simulink model "Transformer_example"  (R2016b)
settings: Solver=VariableStepAuto  StartTime=0.0  StopTime=1000  RelTol=1e-3
InitFcn:
  | d1=1;
  | d2=1;
  | d3=3;
  | d4=3;
  | tau=1000000000000
undefined symbols (not defined in the file): d10, d9
libraries: simulink x1
settings Model: Creator=SHAAD  LastModifiedBy=SHAAD

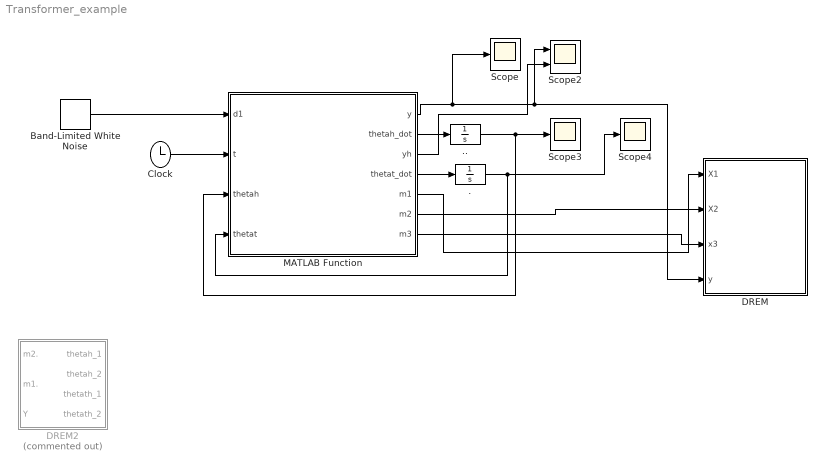
== system Transformer_example ==
  . : Integrator  InitialCondition=[1 2 3]
  .. : Integrator
  Band-Limited White Noise : simulink/Sources/Band-Limited White Noise  Cov=[0.001]  Ts=0.1  seed=[23341]
  Clock : Clock
  DREM : Subsystem
  DREM2 : Subsystem  Commented=on
  MATLAB Function : MATLAB Function  TreatAsAtomicUnit=on
  Scope : Scope
  Scope2 : Scope  NumInputPorts=2
  Scope3 : Scope
  Scope4 : Scope
  wires:
  Clock/1 -> MATLAB Function/2(t)
  MATLAB Function/2(thetah_dot) -> ../1
  ../1 -> MATLAB Function/3(thetah), Scope3/1
  MATLAB Function/4(thetat_dot) -> ./1
  ./1 -> Scope4/1, MATLAB Function/4(thetat)
  MATLAB Function/3(yh) -> Scope2/2
  MATLAB Function/5(m1) -> DREM/1(X1)
  MATLAB Function/6(m2) -> DREM/2(X2)
  MATLAB Function/1(y) -> Scope/1, DREM/4(y), Scope2/1
  MATLAB Function/7(m3) -> DREM/3(x3)
  Band-Limited White Noise/1 -> MATLAB Function/1(d1)

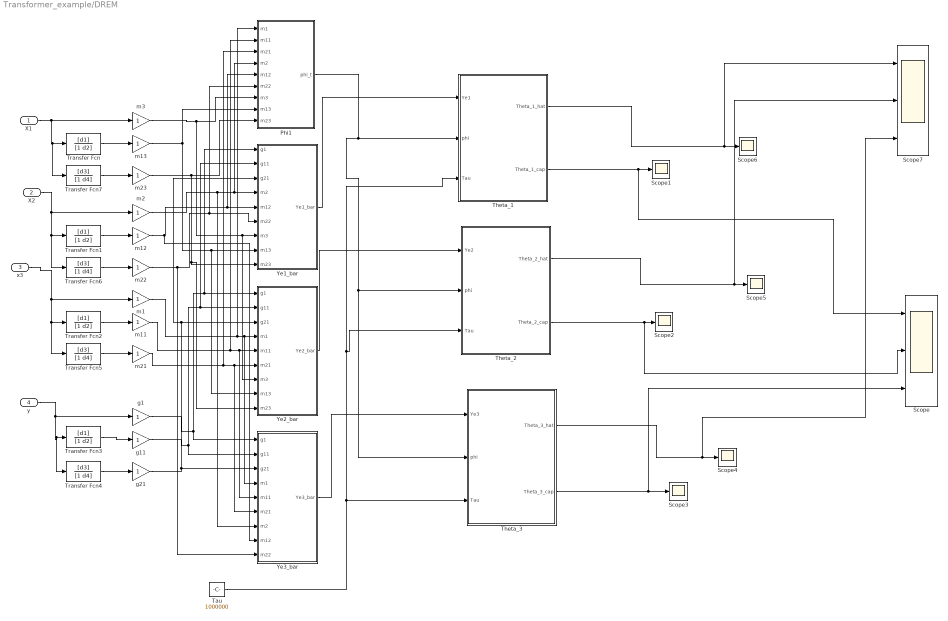
== system Transformer_example/DREM ==
  X1 : Inport
  X2 : Inport  Port=2
  x3 : Inport  Port=3
  y : Inport  Port=4
  Phi1 : Subsystem
  Scope : Scope  NumInputPorts=3
  Scope{1..6} (6 alike) : Scope
  Scope7 : Scope  NumInputPorts=3
  Tau : Constant  Value=1000000  SampleTime=-1
  Theta_1 : Subsystem
  Theta_2 : Subsystem
  Theta_3 : Subsystem
  Transfer Fcn{,1..3} (4 alike) : TransferFcn  Numerator=[d1]  Denominator=[1 d2]
  Transfer Fcn{4..7} (4 alike) : TransferFcn  Numerator=[d3]  Denominator=[1 d4]
  Ye1_bar : Subsystem
  Ye2_bar : Subsystem
  "Ye3_bar " : Subsystem
  g1 : Gain
  g11 : Gain
  g21 : Gain
  m{1..3,11..13,21..23} (9 alike) : Gain
  wires:
  Transfer Fcn/1 -> m13/1
  X1/1 -> m3/1, Transfer Fcn7/1, Transfer Fcn/1
  Transfer Fcn7/1 -> m23/1
  Transfer Fcn1/1 -> m12/1
  X2/1 -> m2/1, Transfer Fcn6/1, Transfer Fcn1/1
  Transfer Fcn6/1 -> m22/1
  x3/1 -> m1/1, Transfer Fcn5/1, Transfer Fcn2/1
  Transfer Fcn5/1 -> m21/1
  Transfer Fcn3/1 -> g11/1
  y/1 -> Transfer Fcn4/1, Transfer Fcn3/1, g1/1
  Transfer Fcn4/1 -> g21/1
  Ye1_bar/1(Ye1_bar) -> Theta_1/1(Ye1)
  Ye2_bar/1(Ye2_bar) -> Theta_2/1(Ye2)
  Phi1/1(phi_t) -> Theta_3/2(phi), Theta_2/2(phi), Theta_1/2(phi)
  Tau/1 -> Theta_3/3(Tau), Theta_2/3(Tau), Theta_1/3(Tau)
  "Ye3_bar "/1(Ye3_bar) -> Theta_3/1(Ye3)
  g1/1 -> Ye1_bar/1(g1), Ye2_bar/1(g1), "Ye3_bar "/1(g1)
  g21/1 -> Ye2_bar/3(g21), Ye1_bar/3(g21), "Ye3_bar "/3(g21)
  m1/1 -> Phi1/1(m1), "Ye3_bar "/4(m1), Ye2_bar/4(m1)
  m11/1 -> Phi1/2(m11), "Ye3_bar "/5(m11), Ye2_bar/5(m11)
  m21/1 -> Phi1/3(m21), "Ye3_bar "/6(m21), Ye2_bar/6(m21)
  m2/1 -> "Ye3_bar "/7(m2), Ye1_bar/4(m2), Phi1/4(m2)
  m12/1 -> "Ye3_bar "/8(m12), Phi1/5(m12), Ye1_bar/5(m12)
  m22/1 -> "Ye3_bar "/9(m22), Ye1_bar/6(m22), Phi1/6(m22)
  m3/1 -> Phi1/7(m3), Ye1_bar/7(m3), Ye2_bar/7(m3)
  m13/1 -> Ye2_bar/8(m13), Ye1_bar/8(m13), Phi1/8(m13)
  m23/1 -> Phi1/9(m23), Ye2_bar/9(m23), Ye1_bar/9(m23)
  Theta_1/1(Theta_1_hat) -> Scope7/1, Scope6/1
  Theta_1/2(Theta_1_cap) -> Scope/1, Scope1/1
  Theta_2/1(Theta_2_hat) -> Scope7/2, Scope5/1
  Theta_2/2(Theta_2_cap) -> Scope/2, Scope2/1
  Theta_3/1(Theta_3_hat) -> Scope7/3, Scope4/1
  Theta_3/2(Theta_3_cap) -> Scope/3, Scope3/1
  Transfer Fcn2/1 -> m11/1
  g11/1 -> Ye1_bar/2(g11), Ye2_bar/2(g11), "Ye3_bar "/2(g11)

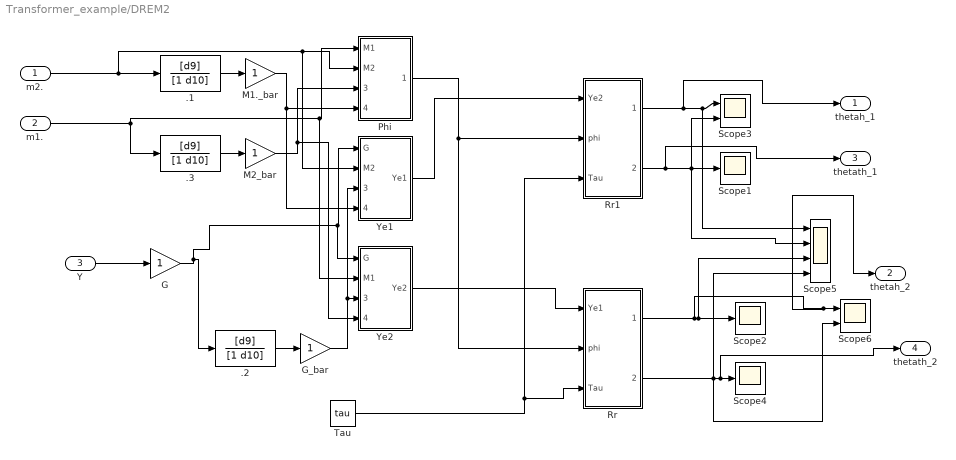
== system Transformer_example/DREM2 ==
  m2. : Inport
  m1. : Inport  Port=2
  Y : Inport  Port=3
  .1 : TransferFcn  Numerator=[d9]  Denominator=[1 d10]
  .2 : TransferFcn  Numerator=[d9]  Denominator=[1 d10]
  .3 : TransferFcn  Numerator=[d9]  Denominator=[1 d10]
  G : Gain
  G_bar : Gain
  M1._bar : Gain
  M2_bar : Gain
  Phi : Subsystem
  Rr : Subsystem
  Rr1 : Subsystem
  Scope1 : Scope
  Scope2 : Scope
  Scope3 : Scope  NumInputPorts=2
  Scope4 : Scope
  Scope5 : Scope  NumInputPorts=4
  Scope6 : Scope  NumInputPorts=2
  Tau : Constant  Value=tau  SampleTime=-1
  Ye1 : Subsystem
  Ye2 : Subsystem
  thetah_1 : Outport
  thetah_2 : Outport  Port=2
  thetath_1 : Outport  Port=3
  thetath_2 : Outport  Port=4
  wires:
  G/1 -> .2/1, Ye2/1(G), Ye1/1(G)
  Tau/1 -> Rr1/3(Tau), Rr/3(Tau)
  Y/1 -> G/1
  .2/1 -> G_bar/1
  .3/1 -> M2_bar/1
  G_bar/1 -> Ye2/3(G_bar), Ye1/3(G_bar)
  Phi/1(phi_t) -> Rr1/2(phi), Rr/2(phi)
  Rr1/2(Rr_cap) -> thetath_1/1, Scope3/2, Scope5/2, Scope1/1
  Rr/1(Rs_hat) -> thetah_2/1, Scope6/1, Scope5/3, Scope2/1
  .1/1 -> M1._bar/1
  Rr1/1(Rr_hat) -> thetah_1/1, Scope5/1, Scope3/1
  m1./1 -> Ye2/2(M1), Phi/1(M1), .3/1
  Ye1/1(Ye1) -> Rr1/1(Ye2)
  Ye2/1(Ye2) -> Rr/1(Ye1)
  M2_bar/1 -> Ye2/4("M1_bar "), Phi/3(M1_bar)
  M1._bar/1 -> Phi/4(M2_bar), Ye1/4(M2_bar)
  m2./1 -> Ye1/2(M2), Phi/2(M2), .1/1
  Rr/2(Rs_cap) -> Scope5/4, Scope6/2, thetath_2/1, Scope4/1

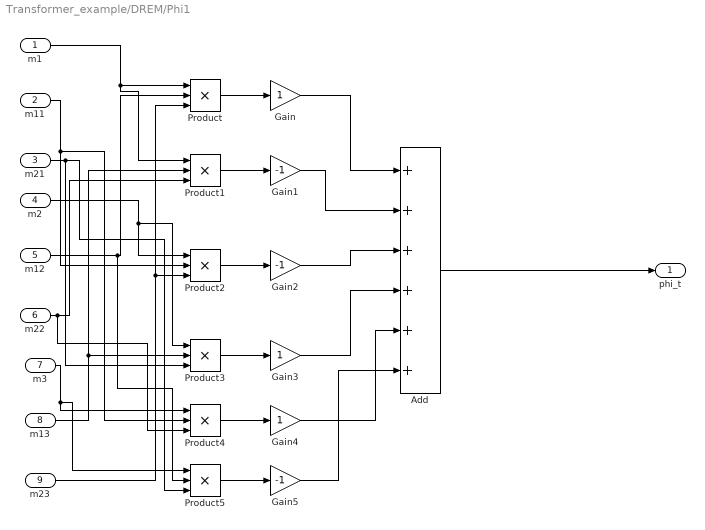
== system Transformer_example/DREM/Phi1 ==
  m1 : Inport
  m11 : Inport  Port=2
  m21 : Inport  Port=3
  m2 : Inport  Port=4
  m12 : Inport  Port=5
  m22 : Inport  Port=6
  m3 : Inport  Port=7
  m13 : Inport  Port=8
  m23 : Inport  Port=9
  Add : Sum  Inputs=++++++
  Gain : Gain
  Gain1 : Gain  Gain=-1
  Gain2 : Gain  Gain=-1
  Gain3 : Gain
  Gain4 : Gain
  Gain5 : Gain  Gain=-1
  Product{,1..5} (6 alike) : Product  Inputs=3
  phi_t : Outport
  wires:
  m1/1 -> Product1/1, Product/1
  m23/1 -> Product2/3, Product/3
  m13/1 -> Product3/2, Product1/2
  m22/1 -> Product4/3, Product1/3
  m2/1 -> Product3/1, Product2/1
  m11/1 -> Product4/2, Product2/2
  m3/1 -> Product5/1, Product4/1
  m12/1 -> Product5/2, Product/2
  m21/1 -> Product5/3, Product3/3
  Product/1 -> Gain/1
  Product1/1 -> Gain1/1
  Product2/1 -> Gain2/1
  Product3/1 -> Gain3/1
  Product4/1 -> Gain4/1
  Product5/1 -> Gain5/1
  Add/1 -> phi_t/1
  Gain/1 -> Add/1
  Gain1/1 -> Add/2
  Gain2/1 -> Add/3
  Gain3/1 -> Add/4
  Gain4/1 -> Add/5
  Gain5/1 -> Add/6

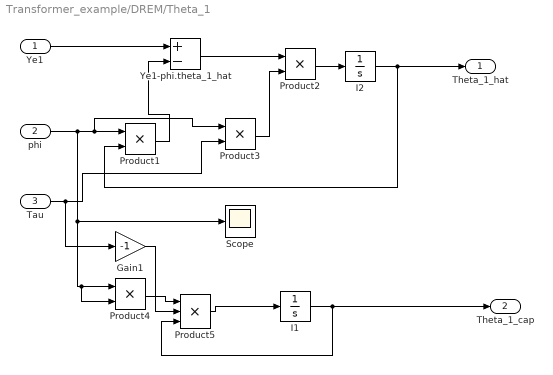
== system Transformer_example/DREM/Theta_1 ==
  Ye1 : Inport
  phi : Inport  Port=2
  Tau : Inport  Port=3
  Gain1 : Gain  Gain=-1
  I1 : Integrator  InitialCondition=1
  I2 : Integrator
  Product{1..4} (4 alike) : Product
  Product5 : Product  Inputs=3
  Scope : Scope
  Ye1-phi.theta_1_hat : Sum  Inputs=+-
  Theta_1_hat : Outport
  Theta_1_cap : Outport  Port=2
  wires:
  Ye1/1 -> Ye1-phi.theta_1_hat/1
  phi/1 -> Scope/1, Product4/2, Product4/1, Product3/1, Product1/1
  Ye1-phi.theta_1_hat/1 -> Product2/1
  Product1/1 -> Ye1-phi.theta_1_hat/2
  Product3/1 -> Product2/2
  Tau/1 -> Gain1/1, Product3/2
  Product2/1 -> I2/1
  Product5/1 -> I1/1
  Product4/1 -> Product5/1
  Gain1/1 -> Product5/2
  I1/1 -> Product5/3, Theta_1_cap/1
  I2/1 -> Product1/2, Theta_1_hat/1

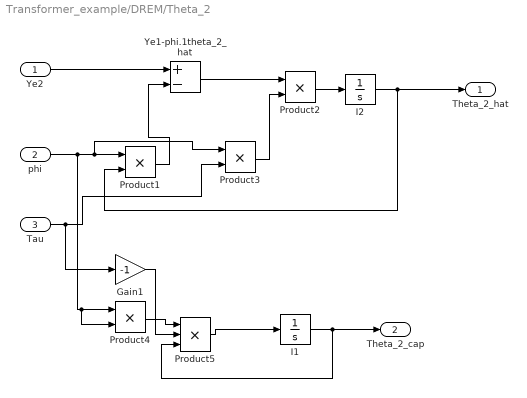
== system Transformer_example/DREM/Theta_2 ==
  Ye2 : Inport
  phi : Inport  Port=2
  Tau : Inport  Port=3
  Gain1 : Gain  Gain=-1
  I1 : Integrator  InitialCondition=-1
  I2 : Integrator
  Product{1..4} (4 alike) : Product
  Product5 : Product  Inputs=3
  Ye1-phi.1theta_2_hat : Sum  Inputs=+-
  Theta_2_hat : Outport
  Theta_2_cap : Outport  Port=2
  wires:
  Ye2/1 -> Ye1-phi.1theta_2_hat/1
  phi/1 -> Product4/2, Product4/1, Product3/1, Product1/1
  Ye1-phi.1theta_2_hat/1 -> Product2/1
  Product1/1 -> Ye1-phi.1theta_2_hat/2
  Product3/1 -> Product2/2
  Tau/1 -> Gain1/1, Product3/2
  Product2/1 -> I2/1
  Product5/1 -> I1/1
  Product4/1 -> Product5/1
  Gain1/1 -> Product5/2
  I1/1 -> Product5/3, Theta_2_cap/1
  I2/1 -> Product1/2, Theta_2_hat/1

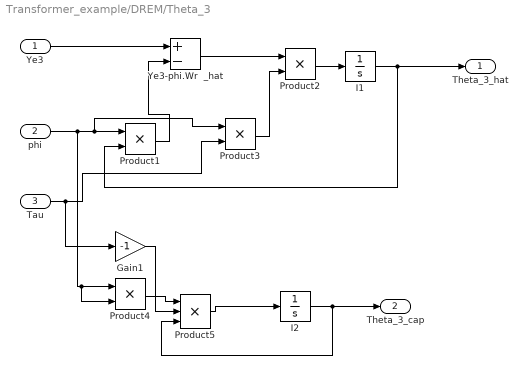
== system Transformer_example/DREM/Theta_3 ==
  Ye3 : Inport
  phi : Inport  Port=2
  Tau : Inport  Port=3
  Gain1 : Gain  Gain=-1
  I1 : Integrator
  I2 : Integrator  InitialCondition=0.5
  Product{1..4} (4 alike) : Product
  Product5 : Product  Inputs=3
  Ye3-phi.Wr  _hat : Sum  Inputs=+-
  Theta_3_hat : Outport
  Theta_3_cap : Outport  Port=2
  wires:
  Ye3/1 -> Ye3-phi.Wr  _hat/1
  phi/1 -> Product4/2, Product4/1, Product3/1, Product1/1
  Ye3-phi.Wr  _hat/1 -> Product2/1
  Product1/1 -> Ye3-phi.Wr  _hat/2
  Product3/1 -> Product2/2
  Tau/1 -> Gain1/1, Product3/2
  Product2/1 -> I1/1
  Product5/1 -> I2/1
  Product4/1 -> Product5/1
  Gain1/1 -> Product5/2
  I2/1 -> Product5/3, Theta_3_cap/1
  I1/1 -> Product1/2, Theta_3_hat/1

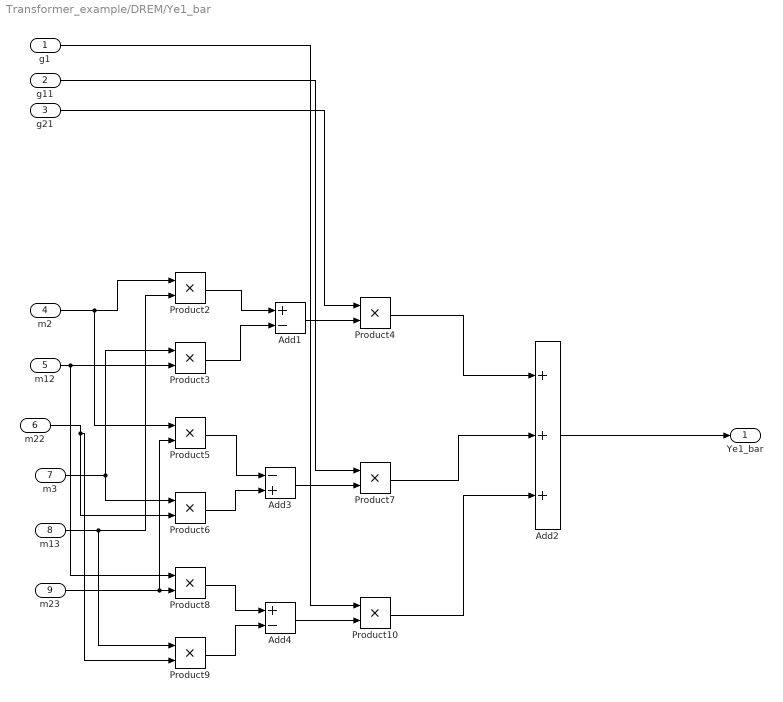
== system Transformer_example/DREM/Ye1_bar ==
  g1 : Inport
  g11 : Inport  Port=2
  g21 : Inport  Port=3
  m2 : Inport  Port=4
  m12 : Inport  Port=5
  m22 : Inport  Port=6
  m3 : Inport  Port=7
  m13 : Inport  Port=8
  m23 : Inport  Port=9
  Add1 : Sum  Inputs=+-
  Add2 : Sum  Inputs=+++
  Add3 : Sum  Inputs=-+
  Add4 : Sum  Inputs=+-
  Product{2..10} (9 alike) : Product
  Ye1_bar : Outport
  wires:
  m2/1 -> Product5/1, Product2/1
  m13/1 -> Product9/1, Product2/2
  m3/1 -> Product6/1, Product3/1
  m12/1 -> Product8/1, Product3/2
  Product2/1 -> Add1/1
  Product3/1 -> Add1/2
  Add1/1 -> Product4/2
  g21/1 -> Product4/1
  Product4/1 -> Add2/1
  m23/1 -> Product8/2, Product5/2
  m22/1 -> Product9/2, Product6/2
  Product5/1 -> Add3/1
  Product6/1 -> Add3/2
  Add3/1 -> Product7/2
  g11/1 -> Product7/1
  Product7/1 -> Add2/2
  Product8/1 -> Add4/1
  Product9/1 -> Add4/2
  Add4/1 -> Product10/2
  g1/1 -> Product10/1
  Product10/1 -> Add2/3
  Add2/1 -> Ye1_bar/1

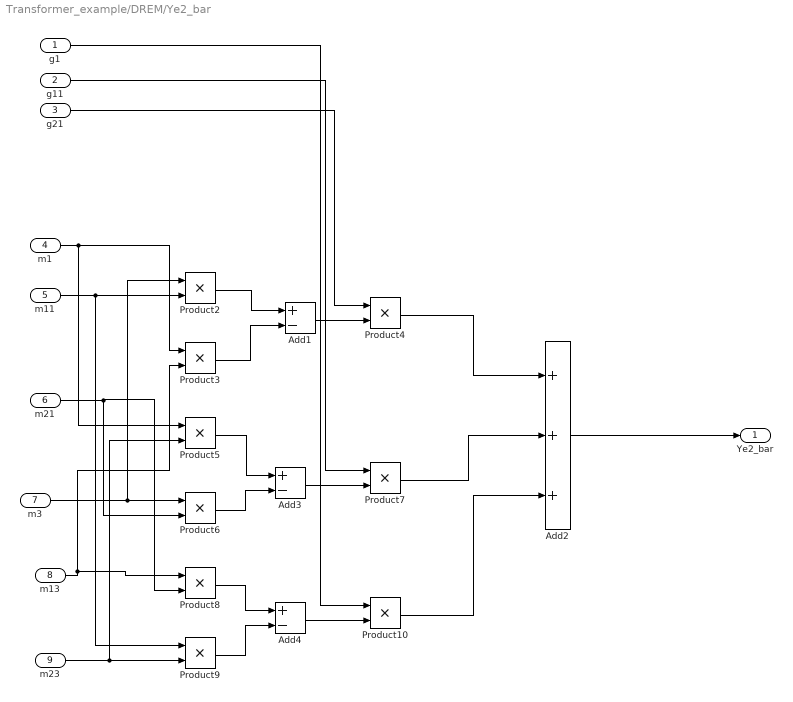
== system Transformer_example/DREM/Ye2_bar ==
  g1 : Inport
  g11 : Inport  Port=2
  g21 : Inport  Port=3
  m1 : Inport  Port=4
  m11 : Inport  Port=5
  m21 : Inport  Port=6
  m3 : Inport  Port=7
  m13 : Inport  Port=8
  m23 : Inport  Port=9
  Add1 : Sum  Inputs=+-
  Add2 : Sum  Inputs=+++
  Add3 : Sum  Inputs=+-
  Add4 : Sum  Inputs=+-
  Product{2..10} (9 alike) : Product
  Ye2_bar : Outport
  wires:
  Product2/1 -> Add1/1
  Product3/1 -> Add1/2
  Add1/1 -> Product4/2
  g21/1 -> Product4/1
  Product4/1 -> Add2/1
  Product5/1 -> Add3/1
  Product6/1 -> Add3/2
  Add3/1 -> Product7/2
  g11/1 -> Product7/1
  Product7/1 -> Add2/2
  Product8/1 -> Add4/1
  Product9/1 -> Add4/2
  Add4/1 -> Product10/2
  g1/1 -> Product10/1
  Product10/1 -> Add2/3
  Add2/1 -> Ye2_bar/1
  m13/1 -> Product3/2, Product8/1
  m21/1 -> Product8/2, Product6/2
  m11/1 -> Product9/1, Product2/2
  m23/1 -> Product5/2, Product9/2
  m1/1 -> Product3/1, Product5/1
  m3/1 -> Product6/1, Product2/1

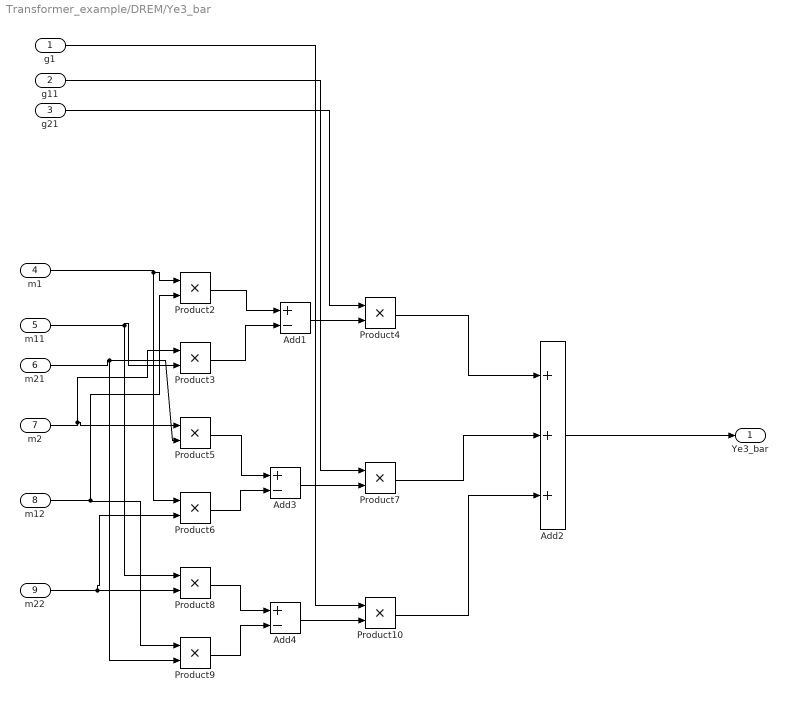
== system Transformer_example/DREM/Ye3_bar  ==
  g1 : Inport
  g11 : Inport  Port=2
  g21 : Inport  Port=3
  m1 : Inport  Port=4
  m11 : Inport  Port=5
  m21 : Inport  Port=6
  m2 : Inport  Port=7
  m12 : Inport  Port=8
  m22 : Inport  Port=9
  Add1 : Sum  Inputs=+-
  Add2 : Sum  Inputs=+++
  Add3 : Sum  Inputs=+-
  Add4 : Sum  Inputs=+-
  Product{2..10} (9 alike) : Product
  Ye3_bar : Outport
  wires:
  Product2/1 -> Add1/1
  Product3/1 -> Add1/2
  Add1/1 -> Product4/2
  g21/1 -> Product4/1
  Product4/1 -> Add2/1
  Product5/1 -> Add3/1
  Product6/1 -> Add3/2
  Add3/1 -> Product7/2
  g11/1 -> Product7/1
  Product7/1 -> Add2/2
  Product8/1 -> Add4/1
  Product9/1 -> Add4/2
  Add4/1 -> Product10/2
  g1/1 -> Product10/1
  Product10/1 -> Add2/3
  Add2/1 -> Ye3_bar/1
  m11/1 -> Product3/2, Product8/1
  m22/1 -> Product6/2, Product8/2
  m12/1 -> Product9/1, Product2/2
  m21/1 -> Product9/2, Product5/2
  m2/1 -> Product3/1, Product5/1
  m1/1 -> Product2/1, Product6/1

== system Transformer_example/DREM2/Phi ==
  M1 : Inport
  M2 : Inport  Port=2
  M1_bar : Inport  Port=3
  M2_bar : Inport  Port=4
  Add : Sum  Inputs=+-
  Product : Product
  Product1 : Product
  phi_t : Outport
  wires:
  M1/1 -> Product/1
  M2_bar/1 -> Product/2
  M2/1 -> Product1/1
  M1_bar/1 -> Product1/2
  Add/1 -> phi_t/1
  Product1/1 -> Add/2
  Product/1 -> Add/1

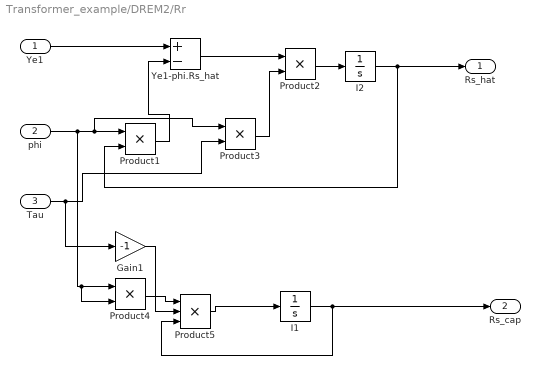
== system Transformer_example/DREM2/Rr ==
  Ye1 : Inport
  phi : Inport  Port=2
  Tau : Inport  Port=3
  Gain1 : Gain  Gain=-1
  I1 : Integrator  InitialCondition=-3
  I2 : Integrator  InitialCondition=0.1
  Product{1..4} (4 alike) : Product
  Product5 : Product  Inputs=3
  Ye1-phi.Rs_hat : Sum  Inputs=+-
  Rs_hat : Outport
  Rs_cap : Outport  Port=2
  wires:
  Ye1/1 -> Ye1-phi.Rs_hat/1
  phi/1 -> Product4/2, Product4/1, Product3/1, Product1/1
  Ye1-phi.Rs_hat/1 -> Product2/1
  Product1/1 -> Ye1-phi.Rs_hat/2
  Product3/1 -> Product2/2
  Tau/1 -> Gain1/1, Product3/2
  Product2/1 -> I2/1
  Product5/1 -> I1/1
  Product4/1 -> Product5/1
  Gain1/1 -> Product5/2
  I1/1 -> Product5/3, Rs_cap/1
  I2/1 -> Product1/2, Rs_hat/1

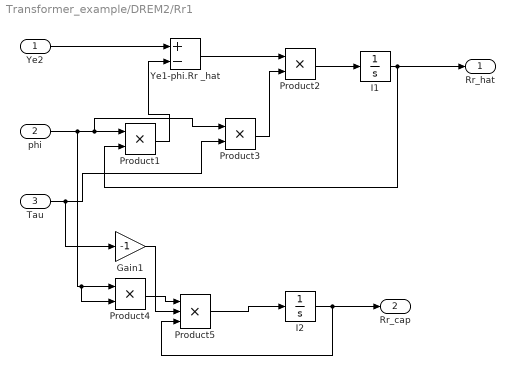
== system Transformer_example/DREM2/Rr1 ==
  Ye2 : Inport
  phi : Inport  Port=2
  Tau : Inport  Port=3
  Gain1 : Gain  Gain=-1
  I1 : Integrator
  I2 : Integrator  InitialCondition=3
  Product{1..4} (4 alike) : Product
  Product5 : Product  Inputs=3
  Ye1-phi.Rr _hat : Sum  Inputs=+-
  Rr_hat : Outport
  Rr_cap : Outport  Port=2
  wires:
  Ye2/1 -> Ye1-phi.Rr _hat/1
  phi/1 -> Product4/2, Product4/1, Product3/1, Product1/1
  Ye1-phi.Rr _hat/1 -> Product2/1
  Product1/1 -> Ye1-phi.Rr _hat/2
  Product3/1 -> Product2/2
  Tau/1 -> Gain1/1, Product3/2
  Product2/1 -> I1/1
  Product5/1 -> I2/1
  Product4/1 -> Product5/1
  Gain1/1 -> Product5/2
  I2/1 -> Product5/3, Rr_cap/1
  I1/1 -> Product1/2, Rr_hat/1

== system Transformer_example/DREM2/Ye1 ==
  G : Inport
  M2 : Inport  Port=2
  G_bar : Inport  Port=3
  M2_bar : Inport  Port=4
  Add : Sum  Inputs=+-
  Product : Product
  Product1 : Product
  Ye1 : Outport
  wires:
  G/1 -> Product/1
  M2_bar/1 -> Product/2
  M2/1 -> Product1/1
  G_bar/1 -> Product1/2
  Add/1 -> Ye1/1
  Product1/1 -> Add/2
  Product/1 -> Add/1

== system Transformer_example/DREM2/Ye2 ==
  G : Inport
  M1 : Inport  Port=2
  G_bar : Inport  Port=3
  "M1_bar " : Inport  Port=4
  Add : Sum
  Gain : Gain  Gain=-1
  Product : Product
  Product1 : Product
  Ye2 : Outport
  wires:
  G/1 -> Product/1
  "M1_bar "/1 -> Product/2
  M1/1 -> Product1/1
  G_bar/1 -> Product1/2
  Add/1 -> Ye2/1
  Product1/1 -> Add/2
  Product/1 -> Gain/1
  Gain/1 -> Add/1

== matlab function Transformer_example/MATLAB Function ==
  data: d1 input; t input; y output; thetah_dot output; yh output; thetat_dot output; m1 output; m2 output; thetah input; thetat input; m3 output
function [y,thetah_dot, yh,  thetat_dot , m1, m2,m3]= fcn(d1,t, thetah, thetat)
M=[d1; sin(t); 1 ];%Regressor
theta=[1;2;3];%Parameter
y = M'*theta;
tau=[1 0 0; 0 1 0; 0 0 1];
thetah_dot=tau*M*(y-M'*thetah);%gradient Estimator
thetat_dot=-tau*M*M'*thetat;
m1=d1;
m2=sin(t);
m3=1;
yh=M'*thetah;
